simulink model "VanDerPol"  (Simulink 7.9)
settings: Solver=ode3  StartTime=0.0  StopTime=10.0  RelTol=1e-3
libraries: simulink x1
settings Model: Creator=Yi  LastModifiedBy=parasara
settings SolverCC: ZeroCrossControl=EnableAll
settings DataIOCC: InitialState=5,5
settings RTWCC: GenCodeOnly=on  TargetLang=C++

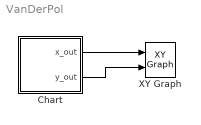
== system VanDerPol ==
  Chart : Stateflow chart  TreatAsAtomicUnit=on
  XY Graph : simulink/Sinks/XY Graph  xmin=-5  xmax=5  ymin=-5  ymax=5  st=0.01
  wires:
  Chart/1(x_out) -> XY Graph/1
  Chart/2(y_out) -> XY Graph/2

== stateflow chart Chart ==
  settings: updateMethod=CONTINUOUS
  state VO
    du:
    x_dot = y;
    y_dot = -y - x - x*x*y;
    x_out = x;
    y_out = y;
  note: @annotation-mode=VO;
      | k=2000;
      | gamma=0;
  (default) -> VO : {x=1.2, y=2.4}
  data: x_out output double; y_out output double; x local double; y local double
  data x settings: updateMethod=SF_CONTINUOUS_TIME_DATA
  data y settings: updateMethod=SF_CONTINUOUS_TIME_DATA
